simulink library "lib_BuildingThermalLiquid"  (R2026a)
settings: Solver=VariableStepAuto
libraries: ExternalWall_lib x47, WallSelector_lib x36, fl_lib x20, RoomWithRadiatorAndUFP x15
(part 2 of 5)

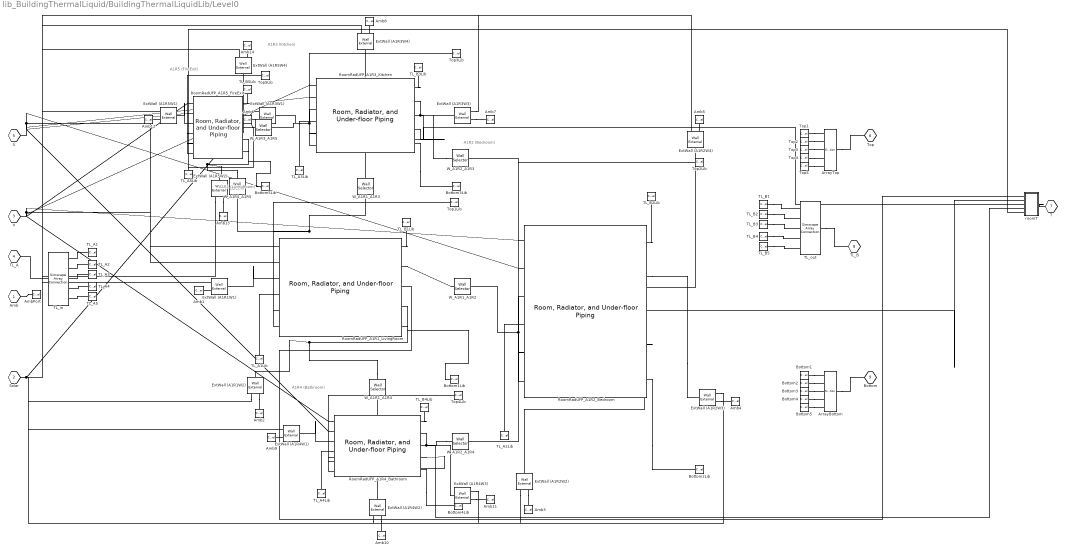
== system lib_BuildingThermalLiquid/BuildingThermalLiquidLib/Level0 ==
  note: A1R1 (LivingRoom)
  note: A1R2 (Bedroom)
  note: A1R3 (Kitchen)
  note: A1R4 (Bathroom)
  note: A1R5 (FireExit)
  Amb{1..14} (14 alike) : ConnectionLabel  Label=A
  AmbPort : ConnectionLabel  Label=A
  ArrayBottom : SimscapeArrayConnection  Domain=foundation.thermal.thermal  ConcatenateDimension=1  NumScalarElements=5
  ArrayTop : SimscapeArrayConnection  Domain=foundation.thermal.thermal  ConcatenateDimension=1  NumScalarElements=5
  Bottom1 : ConnectionLabel  Label=Bottom1
  Bottom1Lib : ConnectionLabel  Label=Bottom1
  Bottom2 : ConnectionLabel  Label=Bottom2
  Bottom2Lib : ConnectionLabel  Label=Bottom2
  Bottom3 : ConnectionLabel  Label=Bottom3
  Bottom3Lib : ConnectionLabel  Label=Bottom3
  Bottom4 : ConnectionLabel  Label=Bottom4
  Bottom4Lib : ConnectionLabel  Label=Bottom4
  Bottom5 : ConnectionLabel  Label=Bottom5
  Bottom5Lib : ConnectionLabel  Label=Bottom5
  ExtWall (A1R1W1) : ExternalWall_lib/Wall External  extWallModel=wallExternalModelOption.wallSolarWin  wallLength=2.4384 % Parameterized on : 11-Dec-2025 09:25:46 m  wallHeight=3.048 % Parameterized on : 11-Dec-2025 09:25:46 m  wallThickness=0.07 % Parameterized on : 11-Dec-2025 09:25:46 m  wallMaterialDen=2000 % Parameterized on : 11-Dec-2025 09:25:47 kg/m^3  wallMaterialCp=1100 % Parameterized on : 11-Dec-2025 09:25:47 J/(K*kg)  wallAbsorptivity=0.6 % Parameterized on : 11-Dec-2025 09:25:47  wallThermalK=1.4 % Parameterized on : 11-Dec-2025 09:25:47 W/(K*m)  winLength=2.0401 % Parameterized on : 11-Dec-2025 09:25:46 m  winHeight=2.5501 % Parameterized on : 11-Dec-2025 09:25:46 m  winThickness=0.005 % Parameterized on : 11-Dec-2025 09:25:47 m  winMaterialDen=4000 % Parameterized on : 11-Dec-2025 09:25:47 kg/m^3  winMaterialCp=840 % Parameterized on : 11-Dec-2025 09:25:47 J/(K*kg)  winAbsorptivity=0.4 % Parameterized on : 11-Dec-2025 09:25:47  winThermalK=1 % Parameterized on : 11-Dec-2025 09:25:47 W/(K*m)  winTransmissivity=0.2 % Parameterized on : 11-Dec-2025 09:25:47  ventLength=0.1 m  ventHeight=0.1 m  extToWallHTC=20 % Parameterized on : 11-Dec-2025 09:25:47 W/(K*m^2)  intToRoomHTC=30 % Parameterized on : 11-Dec-2025 09:25:47 W/(K*m^2)  iniT=300 % Parameterized on : 11-Dec-2025 09:25:47 K  latitude=5  longitude=5  localTime=5  dayLightS=0  surfAngle=90 % Parameterized on : 11-Dec-2025 09:25:46 deg  surfUnitV="[-0.96593    -0.25882] % Parameterized on : 11-Dec-2025 09:25:46"  startYear=2025  startMonth=1  startDay=1  startHr=1  numHrsData=24  interp_method=simscape.enum.interpolation.linear  extrap_method=simscape.enum.extrapolation.nearest
  ExtWall (A1R1W2) : ExternalWall_lib/Wall External  extWallModel=wallExternalModelOption.wallSolarWin  wallLength=3.048 % Parameterized on : 11-Dec-2025 09:25:46 m  wallHeight=3.048 % Parameterized on : 11-Dec-2025 09:25:46 m  wallThickness=0.07 % Parameterized on : 11-Dec-2025 09:25:46 m  wallMaterialDen=2000 % Parameterized on : 11-Dec-2025 09:25:47 kg/m^3  wallMaterialCp=1100 % Parameterized on : 11-Dec-2025 09:25:47 J/(K*kg)  wallAbsorptivity=0.6 % Parameterized on : 11-Dec-2025 09:25:47  wallThermalK=1.4 % Parameterized on : 11-Dec-2025 09:25:47 W/(K*m)  winLength=2.1552 % Parameterized on : 11-Dec-2025 09:25:46 m  winHeight=2.1553 % Parameterized on : 11-Dec-2025 09:25:46 m  winThickness=0.005 % Parameterized on : 11-Dec-2025 09:25:47 m  winMaterialDen=4000 % Parameterized on : 11-Dec-2025 09:25:47 kg/m^3  winMaterialCp=840 % Parameterized on : 11-Dec-2025 09:25:47 J/(K*kg)  winAbsorptivity=0.4 % Parameterized on : 11-Dec-2025 09:25:47  winThermalK=1 % Parameterized on : 11-Dec-2025 09:25:47 W/(K*m)  winTransmissivity=0.2 % Parameterized on : 11-Dec-2025 09:25:47  ventLength=0.1 m  ventHeight=0.1 m  extToWallHTC=20 % Parameterized on : 11-Dec-2025 09:25:47 W/(K*m^2)  intToRoomHTC=30 % Parameterized on : 11-Dec-2025 09:25:47 W/(K*m^2)  iniT=300 % Parameterized on : 11-Dec-2025 09:25:47 K  latitude=5  longitude=5  localTime=5  dayLightS=0  surfAngle=90 % Parameterized on : 11-Dec-2025 09:25:46 deg  surfUnitV="[-0.25882     0.96593] % Parameterized on : 11-Dec-2025 09:25:46"  startYear=2025  startMonth=1  startDay=1  startHr=1  numHrsData=24  interp_method=simscape.enum.interpolation.linear  extrap_method=simscape.enum.extrapolation.nearest
  ExtWall (A1R2W2) : ExternalWall_lib/Wall External  extWallModel=wallExternalModelOption.wallSolar  wallLength=3.048 % Parameterized on : 11-Dec-2025 09:25:46 m  wallHeight=3.048 % Parameterized on : 11-Dec-2025 09:25:46 m  wallThickness=0.07 % Parameterized on : 11-Dec-2025 09:25:46 m  wallMaterialDen=2000 % Parameterized on : 11-Dec-2025 09:25:47 kg/m^3  wallMaterialCp=1100 % Parameterized on : 11-Dec-2025 09:25:47 J/(K*kg)  wallAbsorptivity=0.6 % Parameterized on : 11-Dec-2025 09:25:47  wallThermalK=1.4 % Parameterized on : 11-Dec-2025 09:25:47 W/(K*m)  winLength=1 m  winHeight=0.5 m  winThickness=0.007 m  winMaterialDen=2500 kg/m^3  winMaterialCp=787 J/(K*kg)  winAbsorptivity=0.35  winThermalK=1 W/(K*m)  winTransmissivity=0.45  ventLength=0.1 m  ventHeight=0.1 m  extToWallHTC=20 % Parameterized on : 11-Dec-2025 09:25:47 W/(K*m^2)  intToRoomHTC=30 % Parameterized on : 11-Dec-2025 09:25:47 W/(K*m^2)  iniT=300 % Parameterized on : 11-Dec-2025 09:25:47 K  latitude=5  longitude=5  localTime=5  dayLightS=0  surfAngle=90 % Parameterized on : 11-Dec-2025 09:25:46 deg  surfUnitV="[-0.25882     0.96593] % Parameterized on : 11-Dec-2025 09:25:46"  startYear=2025  startMonth=1  startDay=1  startHr=1  numHrsData=24  interp_method=simscape.enum.interpolation.linear  extrap_method=simscape.enum.extrapolation.nearest
  ExtWall (A1R2W3) : ExternalWall_lib/Wall External  extWallModel=wallExternalModelOption.wallSolarWin  wallLength=4.2672 % Parameterized on : 11-Dec-2025 09:25:46 m  wallHeight=3.048 % Parameterized on : 11-Dec-2025 09:25:46 m  wallThickness=0.07 % Parameterized on : 11-Dec-2025 09:25:46 m  wallMaterialDen=2000 % Parameterized on : 11-Dec-2025 09:25:47 kg/m^3  wallMaterialCp=1100 % Parameterized on : 11-Dec-2025 09:25:47 J/(K*kg)  wallAbsorptivity=0.6 % Parameterized on : 11-Dec-2025 09:25:47  wallThermalK=1.4 % Parameterized on : 11-Dec-2025 09:25:47 W/(K*m)  winLength=3.5702 % Parameterized on : 11-Dec-2025 09:25:46 m  winHeight=2.5501 % Parameterized on : 11-Dec-2025 09:25:46 m  winThickness=0.005 % Parameterized on : 11-Dec-2025 09:25:47 m  winMaterialDen=4000 % Parameterized on : 11-Dec-2025 09:25:47 kg/m^3  winMaterialCp=840 % Parameterized on : 11-Dec-2025 09:25:47 J/(K*kg)  winAbsorptivity=0.4 % Parameterized on : 11-Dec-2025 09:25:47  winThermalK=1 % Parameterized on : 11-Dec-2025 09:25:47 W/(K*m)  winTransmissivity=0.2 % Parameterized on : 11-Dec-2025 09:25:47  ventLength=0.1 m  ventHeight=0.1 m  extToWallHTC=20 % Parameterized on : 11-Dec-2025 09:25:47 W/(K*m^2)  intToRoomHTC=30 % Parameterized on : 11-Dec-2025 09:25:47 W/(K*m^2)  iniT=300 % Parameterized on : 11-Dec-2025 09:25:47 K  latitude=5  longitude=5  localTime=5  dayLightS=0  surfAngle=90 % Parameterized on : 11-Dec-2025 09:25:46 deg  surfUnitV="[0.96593     0.25882] % Parameterized on : 11-Dec-2025 09:25:46"  startYear=2025  startMonth=1  startDay=1  startHr=1  numHrsData=24  interp_method=simscape.enum.interpolation.linear  extrap_method=simscape.enum.extrapolation.nearest
  ExtWall (A1R2W4) : ExternalWall_lib/Wall External  extWallModel=wallExternalModelOption.wallSolarWin  wallLength=3.048 % Parameterized on : 11-Dec-2025 09:25:46 m  wallHeight=3.048 % Parameterized on : 11-Dec-2025 09:25:46 m  wallThickness=0.07 % Parameterized on : 11-Dec-2025 09:25:46 m  wallMaterialDen=2000 % Parameterized on : 11-Dec-2025 09:25:47 kg/m^3  wallMaterialCp=1100 % Parameterized on : 11-Dec-2025 09:25:47 J/(K*kg)  wallAbsorptivity=0.6 % Parameterized on : 11-Dec-2025 09:25:47  wallThermalK=1.4 % Parameterized on : 11-Dec-2025 09:25:47 W/(K*m)  winLength=2.1552 % Parameterized on : 11-Dec-2025 09:25:46 m  winHeight=2.1553 % Parameterized on : 11-Dec-2025 09:25:46 m  winThickness=0.005 % Parameterized on : 11-Dec-2025 09:25:47 m  winMaterialDen=4000 % Parameterized on : 11-Dec-2025 09:25:47 kg/m^3  winMaterialCp=840 % Parameterized on : 11-Dec-2025 09:25:47 J/(K*kg)  winAbsorptivity=0.4 % Parameterized on : 11-Dec-2025 09:25:47  winThermalK=1 % Parameterized on : 11-Dec-2025 09:25:47 W/(K*m)  winTransmissivity=0.2 % Parameterized on : 11-Dec-2025 09:25:47  ventLength=0.1 m  ventHeight=0.1 m  extToWallHTC=20 % Parameterized on : 11-Dec-2025 09:25:47 W/(K*m^2)  intToRoomHTC=30 % Parameterized on : 11-Dec-2025 09:25:47 W/(K*m^2)  iniT=300 % Parameterized on : 11-Dec-2025 09:25:47 K  latitude=5  longitude=5  localTime=5  dayLightS=0  surfAngle=90 % Parameterized on : 11-Dec-2025 09:25:46 deg  surfUnitV="[0.25882    -0.96593] % Parameterized on : 11-Dec-2025 09:25:46"  startYear=2025  startMonth=1  startDay=1  startHr=1  numHrsData=24  interp_method=simscape.enum.interpolation.linear  extrap_method=simscape.enum.extrapolation.nearest
  ExtWall (A1R3W1) : ExternalWall_lib/Wall External  extWallModel=wallExternalModelOption.wallSolar  wallLength=1.8288 % Parameterized on : 11-Dec-2025 09:25:46 m  wallHeight=3.048 % Parameterized on : 11-Dec-2025 09:25:46 m  wallThickness=0.07 % Parameterized on : 11-Dec-2025 09:25:46 m  wallMaterialDen=2000 % Parameterized on : 11-Dec-2025 09:25:47 kg/m^3  wallMaterialCp=1100 % Parameterized on : 11-Dec-2025 09:25:47 J/(K*kg)  wallAbsorptivity=0.6 % Parameterized on : 11-Dec-2025 09:25:47  wallThermalK=1.4 % Parameterized on : 11-Dec-2025 09:25:47 W/(K*m)  winLength=1 m  winHeight=0.5 m  winThickness=0.007 m  winMaterialDen=2500 kg/m^3  winMaterialCp=787 J/(K*kg)  winAbsorptivity=0.35  winThermalK=1 W/(K*m)  winTransmissivity=0.45  ventLength=0.1 m  ventHeight=0.1 m  extToWallHTC=20 % Parameterized on : 11-Dec-2025 09:25:47 W/(K*m^2)  intToRoomHTC=30 % Parameterized on : 11-Dec-2025 09:25:47 W/(K*m^2)  iniT=300 % Parameterized on : 11-Dec-2025 09:25:47 K  latitude=5  longitude=5  localTime=5  dayLightS=0  surfAngle=90 % Parameterized on : 11-Dec-2025 09:25:46 deg  surfUnitV="[-0.96593    -0.25882] % Parameterized on : 11-Dec-2025 09:25:46"  startYear=2025  startMonth=1  startDay=1  startHr=1  numHrsData=24  interp_method=simscape.enum.interpolation.linear  extrap_method=simscape.enum.extrapolation.nearest
  ExtWall (A1R3W3) : ExternalWall_lib/Wall External  extWallModel=wallExternalModelOption.wallSolarWin  wallLength=1.8289 % Parameterized on : 11-Dec-2025 09:25:46 m  wallHeight=3.048 % Parameterized on : 11-Dec-2025 09:25:46 m  wallThickness=0.07 % Parameterized on : 11-Dec-2025 09:25:46 m  wallMaterialDen=2000 % Parameterized on : 11-Dec-2025 09:25:47 kg/m^3  wallMaterialCp=1100 % Parameterized on : 11-Dec-2025 09:25:47 J/(K*kg)  wallAbsorptivity=0.6 % Parameterized on : 11-Dec-2025 09:25:47  wallThermalK=1.4 % Parameterized on : 11-Dec-2025 09:25:47 W/(K*m)  winLength=1.5301 % Parameterized on : 11-Dec-2025 09:25:46 m  winHeight=2.5501 % Parameterized on : 11-Dec-2025 09:25:46 m  winThickness=0.005 % Parameterized on : 11-Dec-2025 09:25:47 m  winMaterialDen=4000 % Parameterized on : 11-Dec-2025 09:25:47 kg/m^3  winMaterialCp=840 % Parameterized on : 11-Dec-2025 09:25:47 J/(K*kg)  winAbsorptivity=0.4 % Parameterized on : 11-Dec-2025 09:25:47  winThermalK=1 % Parameterized on : 11-Dec-2025 09:25:47 W/(K*m)  winTransmissivity=0.2 % Parameterized on : 11-Dec-2025 09:25:47  ventLength=0.1 m  ventHeight=0.1 m  extToWallHTC=20 % Parameterized on : 11-Dec-2025 09:25:47 W/(K*m^2)  intToRoomHTC=30 % Parameterized on : 11-Dec-2025 09:25:47 W/(K*m^2)  iniT=300 % Parameterized on : 11-Dec-2025 09:25:47 K  latitude=5  longitude=5  localTime=5  dayLightS=0  surfAngle=90 % Parameterized on : 11-Dec-2025 09:25:46 deg  surfUnitV="[0.96593     0.25882] % Parameterized on : 11-Dec-2025 09:25:46"  startYear=2025  startMonth=1  startDay=1  startHr=1  numHrsData=24  interp_method=simscape.enum.interpolation.linear  extrap_method=simscape.enum.extrapolation.nearest
  ExtWall (A1R3W4) : ExternalWall_lib/Wall External  extWallModel=wallExternalModelOption.wallSolarWin  wallLength=2.4385 % Parameterized on : 11-Dec-2025 09:25:46 m  wallHeight=3.048 % Parameterized on : 11-Dec-2025 09:25:46 m  wallThickness=0.07 % Parameterized on : 11-Dec-2025 09:25:46 m  wallMaterialDen=2000 % Parameterized on : 11-Dec-2025 09:25:47 kg/m^3  wallMaterialCp=1100 % Parameterized on : 11-Dec-2025 09:25:47 J/(K*kg)  wallAbsorptivity=0.6 % Parameterized on : 11-Dec-2025 09:25:47  wallThermalK=1.4 % Parameterized on : 11-Dec-2025 09:25:47 W/(K*m)  winLength=2.0402 % Parameterized on : 11-Dec-2025 09:25:46 m  winHeight=2.5501 % Parameterized on : 11-Dec-2025 09:25:46 m  winThickness=0.005 % Parameterized on : 11-Dec-2025 09:25:47 m  winMaterialDen=4000 % Parameterized on : 11-Dec-2025 09:25:47 kg/m^3  winMaterialCp=840 % Parameterized on : 11-Dec-2025 09:25:47 J/(K*kg)  winAbsorptivity=0.4 % Parameterized on : 11-Dec-2025 09:25:47  winThermalK=1 % Parameterized on : 11-Dec-2025 09:25:47 W/(K*m)  winTransmissivity=0.2 % Parameterized on : 11-Dec-2025 09:25:47  ventLength=0.1 m  ventHeight=0.1 m  extToWallHTC=20 % Parameterized on : 11-Dec-2025 09:25:47 W/(K*m^2)  intToRoomHTC=30 % Parameterized on : 11-Dec-2025 09:25:47 W/(K*m^2)  iniT=300 % Parameterized on : 11-Dec-2025 09:25:47 K  latitude=5  longitude=5  localTime=5  dayLightS=0  surfAngle=90 % Parameterized on : 11-Dec-2025 09:25:46 deg  surfUnitV="[0.25882    -0.96593] % Parameterized on : 11-Dec-2025 09:25:46"  startYear=2025  startMonth=1  startDay=1  startHr=1  numHrsData=24  interp_method=simscape.enum.interpolation.linear  extrap_method=simscape.enum.extrapolation.nearest
  ExtWall (A1R4W1) : ExternalWall_lib/Wall External  extWallModel=wallExternalModelOption.wallSolar  wallLength=1.524 % Parameterized on : 11-Dec-2025 09:25:46 m  wallHeight=3.048 % Parameterized on : 11-Dec-2025 09:25:46 m  wallThickness=0.07 % Parameterized on : 11-Dec-2025 09:25:46 m  wallMaterialDen=2000 % Parameterized on : 11-Dec-2025 09:25:47 kg/m^3  wallMaterialCp=1100 % Parameterized on : 11-Dec-2025 09:25:47 J/(K*kg)  wallAbsorptivity=0.6 % Parameterized on : 11-Dec-2025 09:25:47  wallThermalK=1.4 % Parameterized on : 11-Dec-2025 09:25:47 W/(K*m)  winLength=1 m  winHeight=0.5 m  winThickness=0.007 m  winMaterialDen=2500 kg/m^3  winMaterialCp=787 J/(K*kg)  winAbsorptivity=0.35  winThermalK=1 W/(K*m)  winTransmissivity=0.45  ventLength=0.1 m  ventHeight=0.1 m  extToWallHTC=20 % Parameterized on : 11-Dec-2025 09:25:47 W/(K*m^2)  intToRoomHTC=30 % Parameterized on : 11-Dec-2025 09:25:47 W/(K*m^2)  iniT=300 % Parameterized on : 11-Dec-2025 09:25:47 K  latitude=5  longitude=5  localTime=5  dayLightS=0  surfAngle=90 % Parameterized on : 11-Dec-2025 09:25:46 deg  surfUnitV="[-0.96593    -0.25882] % Parameterized on : 11-Dec-2025 09:25:46"  startYear=2025  startMonth=1  startDay=1  startHr=1  numHrsData=24  interp_method=simscape.enum.interpolation.linear  extrap_method=simscape.enum.extrapolation.nearest
  ExtWall (A1R4W2) : ExternalWall_lib/Wall External  extWallModel=wallExternalModelOption.wallSolarWin  wallLength=2.1336 % Parameterized on : 11-Dec-2025 09:25:46 m  wallHeight=3.048 % Parameterized on : 11-Dec-2025 09:25:46 m  wallThickness=0.07 % Parameterized on : 11-Dec-2025 09:25:46 m  wallMaterialDen=2000 % Parameterized on : 11-Dec-2025 09:25:47 kg/m^3  wallMaterialCp=1100 % Parameterized on : 11-Dec-2025 09:25:47 J/(K*kg)  wallAbsorptivity=0.6 % Parameterized on : 11-Dec-2025 09:25:47  wallThermalK=1.4 % Parameterized on : 11-Dec-2025 09:25:47 W/(K*m)  winLength=1.1686 % Parameterized on : 11-Dec-2025 09:25:46 m  winHeight=1.6695 % Parameterized on : 11-Dec-2025 09:25:46 m  winThickness=0.005 % Parameterized on : 11-Dec-2025 09:25:47 m  winMaterialDen=4000 % Parameterized on : 11-Dec-2025 09:25:47 kg/m^3  winMaterialCp=840 % Parameterized on : 11-Dec-2025 09:25:47 J/(K*kg)  winAbsorptivity=0.4 % Parameterized on : 11-Dec-2025 09:25:47  winThermalK=1 % Parameterized on : 11-Dec-2025 09:25:47 W/(K*m)  winTransmissivity=0.2 % Parameterized on : 11-Dec-2025 09:25:47  ventLength=0.1 m  ventHeight=0.1 m  extToWallHTC=20 % Parameterized on : 11-Dec-2025 09:25:47 W/(K*m^2)  intToRoomHTC=30 % Parameterized on : 11-Dec-2025 09:25:47 W/(K*m^2)  iniT=300 % Parameterized on : 11-Dec-2025 09:25:47 K  latitude=5  longitude=5  localTime=5  dayLightS=0  surfAngle=90 % Parameterized on : 11-Dec-2025 09:25:46 deg  surfUnitV="[-0.25882     0.96593] % Parameterized on : 11-Dec-2025 09:25:46"  startYear=2025  startMonth=1  startDay=1  startHr=1  numHrsData=24  interp_method=simscape.enum.interpolation.linear  extrap_method=simscape.enum.extrapolation.nearest
  ExtWall (A1R4W3) : ExternalWall_lib/Wall External  extWallModel=wallExternalModelOption.wallSolar  wallLength=1.524 % Parameterized on : 11-Dec-2025 09:25:46 m  wallHeight=3.048 % Parameterized on : 11-Dec-2025 09:25:46 m  wallThickness=0.07 % Parameterized on : 11-Dec-2025 09:25:46 m  wallMaterialDen=2000 % Parameterized on : 11-Dec-2025 09:25:47 kg/m^3  wallMaterialCp=1100 % Parameterized on : 11-Dec-2025 09:25:47 J/(K*kg)  wallAbsorptivity=0.6 % Parameterized on : 11-Dec-2025 09:25:47  wallThermalK=1.4 % Parameterized on : 11-Dec-2025 09:25:47 W/(K*m)  winLength=1 m  winHeight=0.5 m  winThickness=0.007 m  winMaterialDen=2500 kg/m^3  winMaterialCp=787 J/(K*kg)  winAbsorptivity=0.35  winThermalK=1 W/(K*m)  winTransmissivity=0.45  ventLength=0.1 m  ventHeight=0.1 m  extToWallHTC=20 % Parameterized on : 11-Dec-2025 09:25:47 W/(K*m^2)  intToRoomHTC=30 % Parameterized on : 11-Dec-2025 09:25:47 W/(K*m^2)  iniT=300 % Parameterized on : 11-Dec-2025 09:25:47 K  latitude=5  longitude=5  localTime=5  dayLightS=0  surfAngle=90 % Parameterized on : 11-Dec-2025 09:25:46 deg  surfUnitV="[0.96593     0.25882] % Parameterized on : 11-Dec-2025 09:25:46"  startYear=2025  startMonth=1  startDay=1  startHr=1  numHrsData=24  interp_method=simscape.enum.interpolation.linear  extrap_method=simscape.enum.extrapolation.nearest
  ExtWall (A1R5W1) : ExternalWall_lib/Wall External  extWallModel=wallExternalModelOption.wallSolar  wallLength=1.524 % Parameterized on : 11-Dec-2025 09:25:46 m  wallHeight=3.048 % Parameterized on : 11-Dec-2025 09:25:46 m  wallThickness=0.07 % Parameterized on : 11-Dec-2025 09:25:46 m  wallMaterialDen=2000 % Parameterized on : 11-Dec-2025 09:25:47 kg/m^3  wallMaterialCp=1100 % Parameterized on : 11-Dec-2025 09:25:47 J/(K*kg)  wallAbsorptivity=0.6 % Parameterized on : 11-Dec-2025 09:25:47  wallThermalK=1.4 % Parameterized on : 11-Dec-2025 09:25:47 W/(K*m)  winLength=1 m  winHeight=0.5 m  winThickness=0.007 m  winMaterialDen=2500 kg/m^3  winMaterialCp=787 J/(K*kg)  winAbsorptivity=0.35  winThermalK=1 W/(K*m)  winTransmissivity=0.45  ventLength=0.1 m  ventHeight=0.1 m  extToWallHTC=20 % Parameterized on : 11-Dec-2025 09:25:47 W/(K*m^2)  intToRoomHTC=30 % Parameterized on : 11-Dec-2025 09:25:47 W/(K*m^2)  iniT=300 % Parameterized on : 11-Dec-2025 09:25:47 K  latitude=5  longitude=5  localTime=5  dayLightS=0  surfAngle=90 % Parameterized on : 11-Dec-2025 09:25:46 deg  surfUnitV="[-0.96593    -0.25882] % Parameterized on : 11-Dec-2025 09:25:46"  startYear=2025  startMonth=1  startDay=1  startHr=1  numHrsData=24  interp_method=simscape.enum.interpolation.linear  extrap_method=simscape.enum.extrapolation.nearest
  ExtWall (A1R5W2) : ExternalWall_lib/Wall External  extWallModel=wallExternalModelOption.wallSolar  wallLength=1.2192 % Parameterized on : 11-Dec-2025 09:25:46 m  wallHeight=3.048 % Parameterized on : 11-Dec-2025 09:25:46 m  wallThickness=0.07 % Parameterized on : 11-Dec-2025 09:25:46 m  wallMaterialDen=2000 % Parameterized on : 11-Dec-2025 09:25:47 kg/m^3  wallMaterialCp=1100 % Parameterized on : 11-Dec-2025 09:25:47 J/(K*kg)  wallAbsorptivity=0.6 % Parameterized on : 11-Dec-2025 09:25:47  wallThermalK=1.4 % Parameterized on : 11-Dec-2025 09:25:47 W/(K*m)  winLength=1 m  winHeight=0.5 m  winThickness=0.007 m  winMaterialDen=2500 kg/m^3  winMaterialCp=787 J/(K*kg)  winAbsorptivity=0.35  winThermalK=1 W/(K*m)  winTransmissivity=0.45  ventLength=0.1 m  ventHeight=0.1 m  extToWallHTC=20 % Parameterized on : 11-Dec-2025 09:25:47 W/(K*m^2)  intToRoomHTC=30 % Parameterized on : 11-Dec-2025 09:25:47 W/(K*m^2)  iniT=300 % Parameterized on : 11-Dec-2025 09:25:47 K  latitude=5  longitude=5  localTime=5  dayLightS=0  surfAngle=90 % Parameterized on : 11-Dec-2025 09:25:46 deg  surfUnitV="[-0.25882     0.96593] % Parameterized on : 11-Dec-2025 09:25:46"  startYear=2025  startMonth=1  startDay=1  startHr=1  numHrsData=24  interp_method=simscape.enum.interpolation.linear  extrap_method=simscape.enum.extrapolation.nearest
  ExtWall (A1R5W4) : ExternalWall_lib/Wall External  extWallModel=wallExternalModelOption.wallSolarWin  wallLength=1.2192 % Parameterized on : 11-Dec-2025 09:25:46 m  wallHeight=3.048 % Parameterized on : 11-Dec-2025 09:25:46 m  wallThickness=0.07 % Parameterized on : 11-Dec-2025 09:25:46 m  wallMaterialDen=2000 % Parameterized on : 11-Dec-2025 09:25:47 kg/m^3  wallMaterialCp=1100 % Parameterized on : 11-Dec-2025 09:25:47 J/(K*kg)  wallAbsorptivity=0.6 % Parameterized on : 11-Dec-2025 09:25:47  wallThermalK=1.4 % Parameterized on : 11-Dec-2025 09:25:47 W/(K*m)  winLength=0.9444 % Parameterized on : 11-Dec-2025 09:25:46 m  winHeight=2.361 % Parameterized on : 11-Dec-2025 09:25:46 m  winThickness=0.005 % Parameterized on : 11-Dec-2025 09:25:47 m  winMaterialDen=4000 % Parameterized on : 11-Dec-2025 09:25:47 kg/m^3  winMaterialCp=840 % Parameterized on : 11-Dec-2025 09:25:47 J/(K*kg)  winAbsorptivity=0.4 % Parameterized on : 11-Dec-2025 09:25:47  winThermalK=1 % Parameterized on : 11-Dec-2025 09:25:47 W/(K*m)  winTransmissivity=0.2 % Parameterized on : 11-Dec-2025 09:25:47  ventLength=0.1 m  ventHeight=0.1 m  extToWallHTC=20 % Parameterized on : 11-Dec-2025 09:25:47 W/(K*m^2)  intToRoomHTC=30 % Parameterized on : 11-Dec-2025 09:25:47 W/(K*m^2)  iniT=300 % Parameterized on : 11-Dec-2025 09:25:47 K  latitude=5  longitude=5  localTime=5  dayLightS=0  surfAngle=90 % Parameterized on : 11-Dec-2025 09:25:46 deg  surfUnitV="[0.25882    -0.96593] % Parameterized on : 11-Dec-2025 09:25:46"  startYear=2025  startMonth=1  startDay=1  startHr=1  numHrsData=24  interp_method=simscape.enum.interpolation.linear  extrap_method=simscape.enum.extrapolation.nearest
  RoomRadUFP_A1R1_LivingRoom : RoomWithRadiatorAndUFP/Room, Radiator, and Under-floor Piping  pipeRoughnessR=1e-6  pipeLenR=387.096 % Parameterized on : 11-Dec-2025 09:25:47  pipeCrossSectionalAreaR=2.5e-05 % Parameterized on : 11-Dec-2025 09:25:47  pipeHydrDiaR=0.005 % Parameterized on : 11-Dec-2025 09:25:47  pipeRoughnessUFP=1e-6  pipeLenUFP=387.096 % Parameterized on : 11-Dec-2025 09:25:47  pipeCrossSectionalAreaUFP=2.5e-05 % Parameterized on : 11-Dec-2025 09:25:47  pipeHydrDiaUFP=0.005 % Parameterized on : 11-Dec-2025 09:25:47  thermalResFloor=1 % Parameterized on : 11-Dec-2025 09:25:47  roomWid=3.048 % Parameterized on : 11-Dec-2025 09:25:46  roomHgt=3.048 % Parameterized on : 11-Dec-2025 09:25:46  roomLen=2.4384 % Parameterized on : 11-Dec-2025 09:25:46  htc=30 % Parameterized on : 11-Dec-2025 09:25:47  iniT=300 % Parameterized on : 11-Dec-2025 09:25:47  indxS=1  indxV=1
  RoomRadUFP_A1R2_Bedroom : RoomWithRadiatorAndUFP/Room, Radiator, and Under-floor Piping  pipeRoughnessR=1e-6  pipeLenR=542.544 % Parameterized on : 11-Dec-2025 09:25:47  pipeCrossSectionalAreaR=2.5e-05 % Parameterized on : 11-Dec-2025 09:25:47  pipeHydrDiaR=0.005 % Parameterized on : 11-Dec-2025 09:25:47  pipeRoughnessUFP=1e-6  pipeLenUFP=542.544 % Parameterized on : 11-Dec-2025 09:25:47  pipeCrossSectionalAreaUFP=2.5e-05 % Parameterized on : 11-Dec-2025 09:25:47  pipeHydrDiaUFP=0.005 % Parameterized on : 11-Dec-2025 09:25:47  thermalResFloor=1 % Parameterized on : 11-Dec-2025 09:25:47  roomWid=3.048 % Parameterized on : 11-Dec-2025 09:25:46  roomHgt=3.048 % Parameterized on : 11-Dec-2025 09:25:46  roomLen=4.2672 % Parameterized on : 11-Dec-2025 09:25:46  htc=30 % Parameterized on : 11-Dec-2025 09:25:47  iniT=300 % Parameterized on : 11-Dec-2025 09:25:47  indxS=2  indxV=2
  RoomRadUFP_A1R3_Kitchen : RoomWithRadiatorAndUFP/Room, Radiator, and Under-floor Piping  pipeRoughnessR=1e-6  pipeLenR=310.896 % Parameterized on : 11-Dec-2025 09:25:47  pipeCrossSectionalAreaR=2.5e-05 % Parameterized on : 11-Dec-2025 09:25:47  pipeHydrDiaR=0.005 % Parameterized on : 11-Dec-2025 09:25:47  pipeRoughnessUFP=1e-6  pipeLenUFP=310.896 % Parameterized on : 11-Dec-2025 09:25:47  pipeCrossSectionalAreaUFP=2.5e-05 % Parameterized on : 11-Dec-2025 09:25:47  pipeHydrDiaUFP=0.005 % Parameterized on : 11-Dec-2025 09:25:47  thermalResFloor=1 % Parameterized on : 11-Dec-2025 09:25:47  roomWid=2.4384 % Parameterized on : 11-Dec-2025 09:25:46  roomHgt=3.048 % Parameterized on : 11-Dec-2025 09:25:46  roomLen=1.8288 % Parameterized on : 11-Dec-2025 09:25:46  htc=30 % Parameterized on : 11-Dec-2025 09:25:47  iniT=300 % Parameterized on : 11-Dec-2025 09:25:47  indxS=3  indxV=3
  RoomRadUFP_A1R4_Bathroom : RoomWithRadiatorAndUFP/Room, Radiator, and Under-floor Piping  pipeRoughnessR=1e-6  pipeLenR=271.272 % Parameterized on : 11-Dec-2025 09:25:47  pipeCrossSectionalAreaR=2.5e-05 % Parameterized on : 11-Dec-2025 09:25:47  pipeHydrDiaR=0.005 % Parameterized on : 11-Dec-2025 09:25:47  pipeRoughnessUFP=1e-6  pipeLenUFP=271.272 % Parameterized on : 11-Dec-2025 09:25:47  pipeCrossSectionalAreaUFP=2.5e-05 % Parameterized on : 11-Dec-2025 09:25:47  pipeHydrDiaUFP=0.005 % Parameterized on : 11-Dec-2025 09:25:47  thermalResFloor=1 % Parameterized on : 11-Dec-2025 09:25:47  roomWid=2.1336 % Parameterized on : 11-Dec-2025 09:25:46  roomHgt=3.048 % Parameterized on : 11-Dec-2025 09:25:46  roomLen=1.524 % Parameterized on : 11-Dec-2025 09:25:46  htc=30 % Parameterized on : 11-Dec-2025 09:25:47  iniT=300 % Parameterized on : 11-Dec-2025 09:25:47  indxS=4  indxV=4
  RoomRadUFP_A1R5_FireExit : RoomWithRadiatorAndUFP/Room, Radiator, and Under-floor Piping  pipeRoughnessR=1e-6  pipeLenR=193.548 % Parameterized on : 11-Dec-2025 09:25:47  pipeCrossSectionalAreaR=2.5e-05 % Parameterized on : 11-Dec-2025 09:25:47  pipeHydrDiaR=0.005 % Parameterized on : 11-Dec-2025 09:25:47  pipeRoughnessUFP=1e-6  pipeLenUFP=193.548 % Parameterized on : 11-Dec-2025 09:25:47  pipeCrossSectionalAreaUFP=2.5e-05 % Parameterized on : 11-Dec-2025 09:25:47  pipeHydrDiaUFP=0.005 % Parameterized on : 11-Dec-2025 09:25:47  thermalResFloor=1 % Parameterized on : 11-Dec-2025 09:25:47  roomWid=1.2192 % Parameterized on : 11-Dec-2025 09:25:46  roomHgt=3.048 % Parameterized on : 11-Dec-2025 09:25:46  roomLen=1.524 % Parameterized on : 11-Dec-2025 09:25:46  htc=30 % Parameterized on : 11-Dec-2025 09:25:47  iniT=300 % Parameterized on : 11-Dec-2025 09:25:47  indxS=5  indxV=5
  TL_A1 : ConnectionLabel  Label=TL_A1
  TL_A1Lib : ConnectionLabel  Label=TL_A1
  TL_A2 : ConnectionLabel  Label=TL_A2
  TL_A2Lib : ConnectionLabel  Label=TL_A2
  TL_A3 : ConnectionLabel  Label=TL_A3
  TL_A3Lib : ConnectionLabel  Label=TL_A3
  TL_A4 : ConnectionLabel  Label=TL_A4
  TL_A4Lib : ConnectionLabel  Label=TL_A4
  TL_A5 : ConnectionLabel  Label=TL_A5
  TL_A5Lib : ConnectionLabel  Label=TL_A5
  TL_B1 : ConnectionLabel  Label=TL_B1
  TL_B1Lib : ConnectionLabel  Label=TL_B1
  TL_B2 : ConnectionLabel  Label=TL_B2
  TL_B2Lib : ConnectionLabel  Label=TL_B2
  TL_B3 : ConnectionLabel  Label=TL_B3
  TL_B3Lib : ConnectionLabel  Label=TL_B3
  TL_B4 : ConnectionLabel  Label=TL_B4
  TL_B4Lib : ConnectionLabel  Label=TL_B4
  TL_B5 : ConnectionLabel  Label=TL_B5
  TL_B5Lib : ConnectionLabel  Label=TL_B5
  TL_in : SimscapeArrayConnection  Domain=foundation.thermal_liquid.thermal_liquid  ConcatenateDimension=1  NumScalarElements=5
  TL_out : SimscapeArrayConnection  Domain=foundation.thermal_liquid.thermal_liquid  ConcatenateDimension=1  NumScalarElements=5
  Top1 : ConnectionLabel  Label=Top1
  Top1Lib : ConnectionLabel  Label=Top1
  Top2 : ConnectionLabel  Label=Top2
  Top2Lib : ConnectionLabel  Label=Top2
  Top3 : ConnectionLabel  Label=Top3
  Top3Lib : ConnectionLabel  Label=Top3
  Top4 : ConnectionLabel  Label=Top4
  Top4Lib : ConnectionLabel  Label=Top4
  Top5 : ConnectionLabel  Label=Top5
  Top5Lib : ConnectionLabel  Label=Top5
  W_A1R1_A1R2 : WallSelector_lib/Wall Selector  optWall=wallModelOption.wallWinVent  wallLength=2.4384 % Parameterized on : 11-Dec-2025 09:25:46 m  wallHeight=3.048 % Parameterized on : 11-Dec-2025 09:25:46 m  wallThickness=0.04 % Parameterized on : 11-Dec-2025 09:25:46 m  wallMaterialDen=650 % Parameterized on : 11-Dec-2025 09:25:49 kg/m^3  wallMaterialCp=1100 % Parameterized on : 11-Dec-2025 09:25:49 J/(K*kg)  wallAbsorptivity=0.5  wallThermalK=1.4 % Parameterized on : 11-Dec-2025 09:25:49 W/(K*m)  winLength=1 m  winHeight=0.5 m  winThickness=0.007 m  winMaterialDen=2500 kg/m^3  winMaterialCp=787 J/(K*kg)  winAbsorptivity=0.35  winThermalK=1 W/(K*m)  winTransmissivity=0.45  ventLength=1.2192 % Parameterized on : 11-Dec-2025 09:25:46 m  ventHeight=1.524 % Parameterized on : 11-Dec-2025 09:25:46 m  extToWallHTC=30 % Parameterized on : 11-Dec-2025 09:25:49 W/(K*m^2)  intToRoomHTC=30 % Parameterized on : 11-Dec-2025 09:25:49 W/(K*m^2)  iniT=300 % Parameterized on : 11-Dec-2025 09:25:49 K
  W_A1R1_A1R3 : WallSelector_lib/Wall Selector  optWall=wallModelOption.wallWinVent  wallLength=2.4383 % Parameterized on : 11-Dec-2025 09:25:46 m  wallHeight=3.048 % Parameterized on : 11-Dec-2025 09:25:46 m  wallThickness=0.04 % Parameterized on : 11-Dec-2025 09:25:46 m  wallMaterialDen=650 % Parameterized on : 11-Dec-2025 09:25:49 kg/m^3  wallMaterialCp=1100 % Parameterized on : 11-Dec-2025 09:25:49 J/(K*kg)  wallAbsorptivity=0.5  wallThermalK=1.4 % Parameterized on : 11-Dec-2025 09:25:49 W/(K*m)  winLength=1 m  winHeight=0.5 m  winThickness=0.007 m  winMaterialDen=2500 kg/m^3  winMaterialCp=787 J/(K*kg)  winAbsorptivity=0.35  winThermalK=1 W/(K*m)  winTransmissivity=0.45  ventLength=1.7242 % Parameterized on : 11-Dec-2025 09:25:46 m  ventHeight=2.1553 % Parameterized on : 11-Dec-2025 09:25:46 m  extToWallHTC=30 % Parameterized on : 11-Dec-2025 09:25:49 W/(K*m^2)  intToRoomHTC=30 % Parameterized on : 11-Dec-2025 09:25:49 W/(K*m^2)  iniT=300 % Parameterized on : 11-Dec-2025 09:25:49 K
  W_A1R1_A1R4 : WallSelector_lib/Wall Selector  optWall=wallModelOption.wallOnly  wallLength=2.1336 % Parameterized on : 11-Dec-2025 09:25:46 m  wallHeight=3.048 % Parameterized on : 11-Dec-2025 09:25:46 m  wallThickness=0.04 % Parameterized on : 11-Dec-2025 09:25:46 m  wallMaterialDen=650 % Parameterized on : 11-Dec-2025 09:25:49 kg/m^3  wallMaterialCp=1100 % Parameterized on : 11-Dec-2025 09:25:49 J/(K*kg)  wallAbsorptivity=0.5  wallThermalK=1.4 % Parameterized on : 11-Dec-2025 09:25:49 W/(K*m)  winLength=1 m  winHeight=0.5 m  winThickness=0.007 m  winMaterialDen=2500 kg/m^3  winMaterialCp=787 J/(K*kg)  winAbsorptivity=0.35  winThermalK=1 W/(K*m)  winTransmissivity=0.45  ventLength=0.1 m  ventHeight=0.1 m  extToWallHTC=30 % Parameterized on : 11-Dec-2025 09:25:49 W/(K*m^2)  intToRoomHTC=30 % Parameterized on : 11-Dec-2025 09:25:49 W/(K*m^2)  iniT=300 % Parameterized on : 11-Dec-2025 09:25:49 K
  W_A1R1_A1R5 : WallSelector_lib/Wall Selector  optWall=wallModelOption.wallWinVent  wallLength=0.60966 % Parameterized on : 11-Dec-2025 09:25:46 m  wallHeight=3.048 % Parameterized on : 11-Dec-2025 09:25:46 m  wallThickness=0.04 % Parameterized on : 11-Dec-2025 09:25:46 m  wallMaterialDen=650 % Parameterized on : 11-Dec-2025 09:25:49 kg/m^3  wallMaterialCp=1100 % Parameterized on : 11-Dec-2025 09:25:49 J/(K*kg)  wallAbsorptivity=0.5  wallThermalK=1.4 % Parameterized on : 11-Dec-2025 09:25:49 W/(K*m)  winLength=1 m  winHeight=0.5 m  winThickness=0.007 m  winMaterialDen=2500 kg/m^3  winMaterialCp=787 J/(K*kg)  winAbsorptivity=0.35  winThermalK=1 W/(K*m)  winTransmissivity=0.45  ventLength=0.4311 % Parameterized on : 11-Dec-2025 09:25:46 m  ventHeight=2.1553 % Parameterized on : 11-Dec-2025 09:25:46 m  extToWallHTC=30 % Parameterized on : 11-Dec-2025 09:25:49 W/(K*m^2)  intToRoomHTC=30 % Parameterized on : 11-Dec-2025 09:25:49 W/(K*m^2)  iniT=300 % Parameterized on : 11-Dec-2025 09:25:49 K
  W_A1R2_A1R3 : WallSelector_lib/Wall Selector  optWall=wallModelOption.wallOnly  wallLength=0.61001 % Parameterized on : 11-Dec-2025 09:25:46 m  wallHeight=3.048 % Parameterized on : 11-Dec-2025 09:25:46 m  wallThickness=0.04 % Parameterized on : 11-Dec-2025 09:25:46 m  wallMaterialDen=650 % Parameterized on : 11-Dec-2025 09:25:49 kg/m^3  wallMaterialCp=1100 % Parameterized on : 11-Dec-2025 09:25:49 J/(K*kg)  wallAbsorptivity=0.5  wallThermalK=1.4 % Parameterized on : 11-Dec-2025 09:25:49 W/(K*m)  winLength=1 m  winHeight=0.5 m  winThickness=0.007 m  winMaterialDen=2500 kg/m^3  winMaterialCp=787 J/(K*kg)  winAbsorptivity=0.35  winThermalK=1 W/(K*m)  winTransmissivity=0.45  ventLength=0.1 m  ventHeight=0.1 m  extToWallHTC=30 % Parameterized on : 11-Dec-2025 09:25:49 W/(K*m^2)  intToRoomHTC=30 % Parameterized on : 11-Dec-2025 09:25:49 W/(K*m^2)  iniT=300 % Parameterized on : 11-Dec-2025 09:25:49 K
  W_A1R2_A1R4 : WallSelector_lib/Wall Selector  optWall=wallModelOption.wallWinVent  wallLength=1.2188 % Parameterized on : 11-Dec-2025 09:25:46 m  wallHeight=3.048 % Parameterized on : 11-Dec-2025 09:25:46 m  wallThickness=0.04 % Parameterized on : 11-Dec-2025 09:25:46 m  wallMaterialDen=650 % Parameterized on : 11-Dec-2025 09:25:49 kg/m^3  wallMaterialCp=1100 % Parameterized on : 11-Dec-2025 09:25:49 J/(K*kg)  wallAbsorptivity=0.5  wallThermalK=1.4 % Parameterized on : 11-Dec-2025 09:25:49 W/(K*m)  winLength=1 m  winHeight=0.5 m  winThickness=0.007 m  winMaterialDen=2500 kg/m^3  winMaterialCp=787 J/(K*kg)  winAbsorptivity=0.35  winThermalK=1 W/(K*m)  winTransmissivity=0.45  ventLength=0.60942 % Parameterized on : 11-Dec-2025 09:25:46 m  ventHeight=1.524 % Parameterized on : 11-Dec-2025 09:25:46 m  extToWallHTC=30 % Parameterized on : 11-Dec-2025 09:25:49 W/(K*m^2)  intToRoomHTC=30 % Parameterized on : 11-Dec-2025 09:25:49 W/(K*m^2)  iniT=300 % Parameterized on : 11-Dec-2025 09:25:49 K
  W_A1R3_A1R5 : WallSelector_lib/Wall Selector  optWall=wallModelOption.wallOnly  wallLength=1.5239 % Parameterized on : 11-Dec-2025 09:25:46 m  wallHeight=3.048 % Parameterized on : 11-Dec-2025 09:25:46 m  wallThickness=0.04 % Parameterized on : 11-Dec-2025 09:25:46 m  wallMaterialDen=650 % Parameterized on : 11-Dec-2025 09:25:49 kg/m^3  wallMaterialCp=1100 % Parameterized on : 11-Dec-2025 09:25:49 J/(K*kg)  wallAbsorptivity=0.5  wallThermalK=1.4 % Parameterized on : 11-Dec-2025 09:25:49 W/(K*m)  winLength=1 m  winHeight=0.5 m  winThickness=0.007 m  winMaterialDen=2500 kg/m^3  winMaterialCp=787 J/(K*kg)  winAbsorptivity=0.35  winThermalK=1 W/(K*m)  winTransmissivity=0.45  ventLength=0.1 m  ventHeight=0.1 m  extToWallHTC=30 % Parameterized on : 11-Dec-2025 09:25:49 W/(K*m^2)  intToRoomHTC=30 % Parameterized on : 11-Dec-2025 09:25:49 W/(K*m^2)  iniT=300 % Parameterized on : 11-Dec-2025 09:25:49 K
  roomT : Subsystem
  Amb : PMIOPort  Side=Left
  Solar : PMIOPort  Port=2  Side=Left
  V : PMIOPort  Port=3  Side=Left
  TL_A : PMIOPort  Port=4  Side=Left
  S : PMIOPort  Port=5  Side=Left
  Top : PMIOPort  Port=6  Side=Left
  T : PMIOPort  Port=7  Side=Right
  TL_B : PMIOPort  Port=8  Side=Right
  Bottom : PMIOPort  Port=9  Side=Right
  connections:
  RoomRadUFP_A1R1_LivingRoom/RConn2 -- W_A1R1_A1R2/RConn1
  W_A1R1_A1R2/LConn1 -- RoomRadUFP_A1R2_Bedroom/LConn3 -- W_A1R2_A1R3/RConn1 -- W_A1R2_A1R4/RConn1
  W_A1R1_A1R3/RConn1 -- RoomRadUFP_A1R1_LivingRoom/LConn5 -- W_A1R1_A1R5/RConn1
  RoomRadUFP_A1R3_Kitchen/RConn4 -- W_A1R1_A1R3/LConn1
  W_A1R1_A1R4/RConn1 -- RoomRadUFP_A1R1_LivingRoom/RConn4 -- ExtWall (A1R1W2)/RConn1
  RoomRadUFP_A1R4_Bathroom/LConn5 -- W_A1R1_A1R4/LConn1
  W_A1R1_A1R5/LConn1 -- RoomRadUFP_A1R5_FireExit/RConn4 -- ExtWall (A1R5W2)/RConn1
  W_A1R2_A1R3/LConn1 -- RoomRadUFP_A1R3_Kitchen/RConn2 -- ExtWall (A1R3W3)/RConn1
  W_A1R2_A1R4/LConn1 -- RoomRadUFP_A1R4_Bathroom/RConn2 -- ExtWall (A1R4W3)/RConn1
  W_A1R3_A1R5/RConn1 -- RoomRadUFP_A1R3_Kitchen/LConn3 -- ExtWall (A1R3W1)/RConn1
  RoomRadUFP_A1R5_FireExit/RConn2 -- W_A1R3_A1R5/LConn1
  RoomRadUFP_A1R1_LivingRoom/LConn3 -- ExtWall (A1R1W1)/RConn1
  ExtWall (A1R1W1)/LConn2 -- Amb1/LConn1
  ExtWall (A1R1W2)/LConn2 -- Amb2/LConn1
  RoomRadUFP_A1R2_Bedroom/RConn4 -- ExtWall (A1R2W2)/RConn1
  ExtWall (A1R2W2)/LConn2 -- Amb3/LConn1
  RoomRadUFP_A1R2_Bedroom/RConn2 -- ExtWall (A1R2W3)/RConn1
  ExtWall (A1R2W3)/LConn2 -- Amb4/LConn1
  RoomRadUFP_A1R2_Bedroom/LConn5 -- ExtWall (A1R2W4)/RConn1
  ExtWall (A1R2W4)/LConn2 -- Amb5/LConn1
  ExtWall (A1R3W1)/LConn2 -- Amb6/LConn1
  ExtWall (A1R3W3)/LConn2 -- Amb7/LConn1
  RoomRadUFP_A1R3_Kitchen/LConn5 -- ExtWall (A1R3W4)/RConn1
  ExtWall (A1R3W4)/LConn2 -- Amb8/LConn1
  RoomRadUFP_A1R4_Bathroom/LConn3 -- ExtWall (A1R4W1)/RConn1
  ExtWall (A1R4W1)/LConn2 -- Amb9/LConn1
  RoomRadUFP_A1R4_Bathroom/RConn4 -- ExtWall (A1R4W2)/RConn1
  ExtWall (A1R4W2)/LConn2 -- Amb10/LConn1
  ExtWall (A1R4W3)/LConn2 -- Amb11/LConn1
  RoomRadUFP_A1R5_FireExit/LConn3 -- ExtWall (A1R5W1)/RConn1
  ExtWall (A1R5W1)/LConn2 -- Amb12/LConn1
  ExtWall (A1R5W2)/LConn2 -- Amb13/LConn1
  RoomRadUFP_A1R5_FireExit/LConn5 -- ExtWall (A1R5W4)/RConn1
  ExtWall (A1R5W4)/LConn2 -- Amb14/LConn1
  Amb/RConn1 -- AmbPort/LConn1
  ExtWall (A1R1W1)/LConn1 -- ExtWall (A1R1W2)/LConn1 -- ExtWall (A1R2W2)/LConn1 -- ExtWall (A1R2W3)/LConn1 -- ExtWall (A1R2W4)/LConn1 -- ExtWall (A1R3W1)/LConn1 -- ExtWall (A1R3W3)/LConn1 -- ExtWall (A1R3W4)/LConn1 -- ExtWall (A1R4W1)/LConn1 -- ExtWall (A1R4W2)/LConn1 -- ExtWall (A1R4W3)/LConn1 -- ExtWall (A1R5W1)/LConn1 -- ExtWall (A1R5W2)/LConn1 -- Solar/RConn1 -- ExtWall (A1R5W4)/LConn1
  roomT/LConn1 -- RoomRadUFP_A1R1_LivingRoom/RConn3
  roomT/LConn2 -- RoomRadUFP_A1R2_Bedroom/RConn3
  roomT/LConn3 -- RoomRadUFP_A1R3_Kitchen/RConn3
  roomT/LConn4 -- RoomRadUFP_A1R4_Bathroom/RConn3
  roomT/LConn5 -- RoomRadUFP_A1R5_FireExit/RConn3
  roomT/RConn1 -- T/RConn1
  TL_A1/LConn1 -- TL_in/LConn1
  TL_A2/LConn1 -- TL_in/LConn2
  TL_A3/LConn1 -- TL_in/LConn3
  TL_A4/LConn1 -- TL_in/LConn4
  TL_A5/LConn1 -- TL_in/LConn5
  TL_in/RConn1 -- TL_A/RConn1
  TL_B1/LConn1 -- TL_out/LConn1
  TL_B2/LConn1 -- TL_out/LConn2
  TL_B3/LConn1 -- TL_out/LConn3
  TL_B4/LConn1 -- TL_out/LConn4
  TL_B5/LConn1 -- TL_out/LConn5
  TL_out/RConn1 -- TL_B/RConn1
  RoomRadUFP_A1R1_LivingRoom/LConn4 -- TL_A1Lib/LConn1
  RoomRadUFP_A1R1_LivingRoom/RConn1 -- TL_B1Lib/LConn1
  RoomRadUFP_A1R2_Bedroom/LConn4 -- TL_A2Lib/LConn1
  RoomRadUFP_A1R2_Bedroom/RConn1 -- TL_B2Lib/LConn1
  RoomRadUFP_A1R3_Kitchen/LConn4 -- TL_A3Lib/LConn1
  RoomRadUFP_A1R3_Kitchen/RConn1 -- TL_B3Lib/LConn1
  RoomRadUFP_A1R4_Bathroom/LConn4 -- TL_A4Lib/LConn1
  RoomRadUFP_A1R4_Bathroom/RConn1 -- TL_B4Lib/LConn1
  RoomRadUFP_A1R5_FireExit/LConn4 -- TL_A5Lib/LConn1
  RoomRadUFP_A1R5_FireExit/RConn1 -- TL_B5Lib/LConn1
  RoomRadUFP_A1R1_LivingRoom/LConn2 -- RoomRadUFP_A1R2_Bedroom/LConn2 -- RoomRadUFP_A1R3_Kitchen/LConn2 -- RoomRadUFP_A1R4_Bathroom/LConn2 -- S/RConn1 -- RoomRadUFP_A1R5_FireExit/LConn2
  RoomRadUFP_A1R1_LivingRoom/LConn1 -- RoomRadUFP_A1R2_Bedroom/LConn1 -- RoomRadUFP_A1R3_Kitchen/LConn1 -- RoomRadUFP_A1R4_Bathroom/LConn1 -- V/RConn1 -- RoomRadUFP_A1R5_FireExit/LConn1
  Top1/LConn1 -- ArrayTop/LConn1
  Top2/LConn1 -- ArrayTop/LConn2
  Top3/LConn1 -- ArrayTop/LConn3
  Top4/LConn1 -- ArrayTop/LConn4
  Top5/LConn1 -- ArrayTop/LConn5
  ArrayTop/RConn1 -- Top/RConn1
  RoomRadUFP_A1R1_LivingRoom/LConn6 -- Top1Lib/LConn1
  RoomRadUFP_A1R2_Bedroom/LConn6 -- Top2Lib/LConn1
  RoomRadUFP_A1R3_Kitchen/LConn6 -- Top3Lib/LConn1
  RoomRadUFP_A1R4_Bathroom/LConn6 -- Top4Lib/LConn1
  RoomRadUFP_A1R5_FireExit/LConn6 -- Top5Lib/LConn1
  Bottom1/LConn1 -- ArrayBottom/LConn1
  Bottom2/LConn1 -- ArrayBottom/LConn2
  Bottom3/LConn1 -- ArrayBottom/LConn3
  Bottom4/LConn1 -- ArrayBottom/LConn4
  Bottom5/LConn1 -- ArrayBottom/LConn5
  ArrayBottom/RConn1 -- Bottom/RConn1
  RoomRadUFP_A1R1_LivingRoom/RConn5 -- Bottom1Lib/LConn1
  RoomRadUFP_A1R2_Bedroom/RConn5 -- Bottom2Lib/LConn1
  RoomRadUFP_A1R3_Kitchen/RConn5 -- Bottom3Lib/LConn1
  RoomRadUFP_A1R4_Bathroom/RConn5 -- Bottom4Lib/LConn1
  RoomRadUFP_A1R5_FireExit/RConn5 -- Bottom5Lib/LConn1
